simulink model "sl_rrmc2"  (Simulink 7.6)
settings: Solver=ode45  StartTime=0.0  StopTime=10.0  RelTol=1e-3
PreLoadFcn:
  | fprintf('*** Loading Puma560 model to workspace\n');
  | mdl_puma560
undefined symbols (not defined in the file or in its folder): DiscIntNeverNeededParam, p560, qn, transl
libraries: roblocks x5, simulink x1
settings Model: Creator=pic  LastModifiedBy=n6334687  ExtModeTrigMode=oneshot  ExtModeArmWhenConnect=off
settings DataIOCC: LimitDataPoints=off
settings OptimizationCC: BlockReduction=off  BooleanDataType=off  InitFltsAndDblsToZero=on
settings DebuggingCC: SaveWithParameterizedLinksMsg=none  SignalResolutionControl=TryResolveAllWithWarning  SolverPrmCheckMsg=none  MultiTaskDSMMsg=warning  MultiTaskCondExecSysMsg=none  StrictBusMsg=None
settings HardwareCC: TargetUnknown=on
settings RTWCC: IncludeERTFirstTime=on
settings GRTTargetCC: ModelReferenceCompliant=off  CompOptLevelCompliant=off  MatFileLogging=off

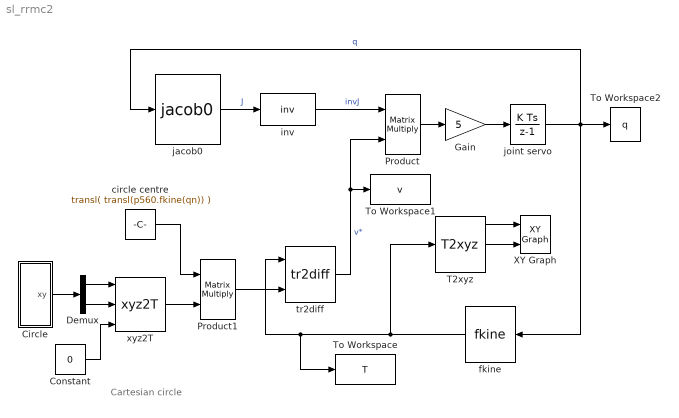
== system sl_rrmc2 ==
  note: Cartesian circle
  Circle : Subsystem  mask{radius=0.05, freq=0.2}
      mask prompts: freq "Frequency (rev/s)"
  Constant : Constant  Value=0
  Demux : Demux  Outputs=2
  Gain : Gain  Gain=5  SaturateOnIntegerOverflow=on  OutDataTypeStr=Inherit: Same as input  ParamDataTypeStr=Inherit: Same as input
  Product : Product  Multiplication=Matrix(*)  SaturateOnIntegerOverflow=on  RndMeth=Zero  InputSameDT=on  OutDataTypeStr=Inherit: Same as first input
  Product1 : Product  Multiplication=Matrix(*)  SaturateOnIntegerOverflow=on  RndMeth=Zero  InputSameDT=on  OutDataTypeStr=Inherit: Same as first input
  T2xyz : roblocks/Transform Conversion/T2xyz  SystemSampleTime=-1
  To Workspace : ToWorkspace  VariableName=T  SampleTime=-1  SaveFormat=Array
  To Workspace1 : ToWorkspace  VariableName=v  SampleTime=-1  SaveFormat=Array
  To Workspace2 : ToWorkspace  VariableName=q  SampleTime=-1  SaveFormat=Array
  XY Graph : simulink/Sinks/XY Graph  SystemSampleTime=-1  xmin=0.5  xmax=0.7  ymin=-0.25  ymax=-0.05  st=-1
  circle centre : Constant  Value=transl( transl(p560.fkine(qn)) )
  fkine : roblocks/Kinematics/fkine  SystemSampleTime=-1  robot=p560
  inv : MATLABFcn  MATLABFcn=inv  Output1D=off
  "jacob0 " : roblocks/Kinematics/jacob0   SystemSampleTime=-1  robot=p560
  joint servo : DiscreteIntegrator  InitialCondition=qn'  SampleTime=0.05  ICPrevOutput=DiscIntNeverNeededParam  ICPrevScaledInput=DiscIntNeverNeededParam
  tr2diff : roblocks/Kinematics/tr2diff  SystemSampleTime=-1  robot=p560
  xyz2T : roblocks/Transform Conversion/xyz2T  SystemSampleTime=-1
  wires:
  joint servo/1 -> "jacob0 "/1, fkine/1, To Workspace2/1  "q"
  T2xyz/1 -> XY Graph/1
  T2xyz/2 -> XY Graph/2
  tr2diff/1 -> Product/2, To Workspace1/1  "v*"
  Demux/1 -> xyz2T/1
  "jacob0 "/1 -> inv/1  "J"
  Product/1 -> Gain/1
  inv/1 -> Product/1  "invJ"
  Gain/1 -> joint servo/1
  Demux/2 -> xyz2T/2
  Circle/1(xy) -> Demux/1
  Constant/1 -> xyz2T/3
  fkine/1 -> T2xyz/1, To Workspace/1, tr2diff/1
  xyz2T/1 -> Product1/2
  circle centre/1 -> Product1/1
  Product1/1 -> tr2diff/2

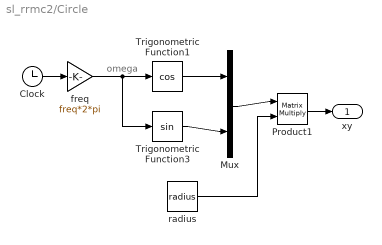
== system sl_rrmc2/Circle ==
  note: omega
  Clock : Clock
      settings: Decimation=10
  Mux : Mux  Inputs=2
  Product1 : Product  Multiplication=Matrix(*)  RndMeth=Zero
  Trigonometric Function1 : Trigonometry  Operator=cos
  Trigonometric Function3 : Trigonometry
  freq : Gain  Gain=freq*2*pi
  radius : Constant  Value=radius
  xy : Outport
  wires:
  freq/1 -> Trigonometric Function3/1, Trigonometric Function1/1
  Product1/1 -> xy/1
  Clock/1 -> freq/1
  radius/1 -> Product1/2
  Mux/1 -> Product1/1
  Trigonometric Function1/1 -> Mux/1
  Trigonometric Function3/1 -> Mux/2
